simulink model "plant"  (R2018b)
settings: Solver=FixedStepAuto  StartTime=0.0  StopTime=10.0  RelTol=1e-3
values from neighbouring files (symbols this model uses):
  A = ((6+5/8)/2)^2    (= 10.97265625)    [setup.m]
  heater_temp = 125    [setup.m]
  pump_rate = 20    [setup.m]
  tank_x0 = 50    [setup.m]
  water_demand = .5    (= 0.5)    [setup.m]
  water_leak = 0    [setup.m]
settings Model: Creator=jayakumarav  LastModifiedBy=hiterd
settings DebuggingCC: LibraryContextMissingDiagnostic=none
settings SFSimCC: SimUseLocalCustomCode=off
settings RTWCC: RTWUseLocalCustomCode=off

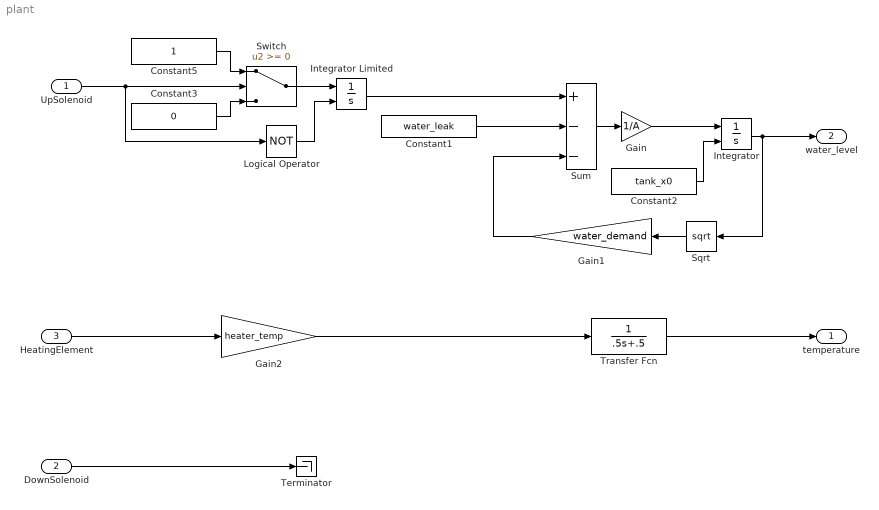
== system plant ==
  UpSolenoid : Inport  OutDataTypeStr=boolean
  DownSolenoid : Inport  Port=2  OutDataTypeStr=boolean
  HeatingElement : Inport  Port=3  OutDataTypeStr=boolean
  Constant1 : Constant  Value=water_leak  SampleTime=-1
  Constant2 : Constant  Value=tank_x0  SampleTime=-1
  Constant3 : Constant  Value=0  SampleTime=-1
  Constant5 : Constant  SampleTime=-1
  Gain : Gain  Gain=1/A
  Gain1 : Gain  Gain=water_demand
  Gain2 : Gain  Gain=heater_temp  OutDataTypeStr=double
  Integrator : Integrator  InitialConditionSource=external
  Integrator Limited : Integrator  ExternalReset=rising  LimitOutput=on  UpperSaturationLimit=pump_rate  LowerSaturationLimit=0
  Logical Operator : Logic  Operator=NOT  AllPortsSameDT=off  OutDataTypeStr=boolean
  Sqrt : Sqrt  SaturateOnIntegerOverflow=on
  Sum : Sum  Inputs=+--
  Switch : Switch
  Terminator : Terminator
  Transfer Fcn : TransferFcn  Denominator=[.5 .5]
  temperature : Outport
  water_level : Outport  Port=2
  wires:
  DownSolenoid/1 -> Terminator/1
  UpSolenoid/1 -> Logical Operator/1, Switch/2
  Sqrt/1 -> Gain1/1
  Constant1/1 -> Sum/2
  Gain1/1 -> Sum/3
  Gain/1 -> Integrator/1
  Sum/1 -> Gain/1
  HeatingElement/1 -> Gain2/1
  Gain2/1 -> Transfer Fcn/1
  Integrator/1 -> Sqrt/1, water_level/1
  Transfer Fcn/1 -> temperature/1
  Constant2/1 -> Integrator/2
  Integrator Limited/1 -> Sum/1
  Constant5/1 -> Switch/1
  Constant3/1 -> Switch/3
  Switch/1 -> Integrator Limited/1
  Logical Operator/1 -> Integrator Limited/2
